simulink model "mpc_onlineHorizons"  (R2023a)
settings: Solver=ode23s  StartTime=0.0  StopTime=10  RelTol=1e-3
values from neighbouring files (symbols this model uses):
  r0 = -0.7    [RunTimeHorizonAdjustment1.m]
  x0 = [op_report.States(1).x;op_report.States(2).x]    [RunTimeHorizonAdjustment1.m]
  y0 = op_report.Outputs.y    [RunTimeHorizonAdjustment1.m]
libraries: mpclib x1
settings Model: ExtModeTrigMode=oneshot  Creator=The MathWorks, Inc.  LastModifiedBy=The MathWorks, Inc.
settings SolverCC: AlgebraicLoopSolver=TrustRegion
settings DataIOCC: SaveFormat=Array  ReturnWorkspaceOutputs=off  SignalLoggingName=sigsOut
settings OptimizationCC: BooleanDataType=off  ExpressionDepthLimit=2147483647  InitFltsAndDblsToZero=on  LifeSpan=inf
settings DebuggingCC: UnderspecifiedInitializationDetection=Classic  MergeDetectMultiDrivingBlocksExec=none  CheckExecutionContextPreStartOutputMsg=on  SignalResolutionControl=TryResolveAllWithWarning  MultiTaskDSMMsg=warning  MultiTaskCondExecSysMsg=none  IntegerOverflowMsg=none  FcnCallInpInsideContextMsg=warning  UnconnectedInputMsg=warning  UnconnectedOutputMsg=warning  UnconnectedLineMsg=warning  StateNameClashWarn=warning  SFUnexpectedBacktrackingDiag=warning  SFNoUnconditionalDefaultTransitionDiag=warning  SFExecutionAtInitializationDiag=none  IntegerSaturationMsg=none  ArithmeticOperatorsInVariantConditions=warning
settings HardwareCC: ProdBitPerPointer=32  ProdBitPerSizeT=32  ProdBitPerPtrDiffT=32  ProdLargestAtomicFloat=None  ProdIntDivRoundTo=Undefined  ProdEndianess=Unspecified  ProdWordSize=32  ProdHWDeviceType=32-bit Generic  TargetUnknown=on
settings ModelReferenceCC: EnableRefExpFcnMdlSchedulingChecks=on  PropagateSignalLabelsOutOfModel=off
settings SFSimCC: SimUseLocalCustomCode=off  CustomCodeUndefinedFunction=UseInterfaceOnly
settings RTWCC: RTWUseLocalCustomCode=off
settings CodeAppCC: StateflowObjectComments=on
settings GRTTargetCC: TargetLangStandard=C89/C90 (ANSI)  CombineOutputUpdateFcns=off  GRTInterface=on
settings ConfigComp: CovMetricSettings=dw  CovSaveCumulativeToWorkspaceVar=on  CovSaveSingleToWorkspaceVar=on  CovExternalEMLEnable=off  CovSFcnEnable=off

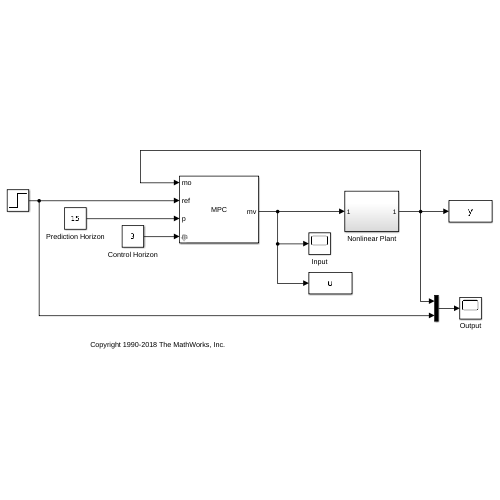
[thumbnail: Simulink's stored preview of the top-level diagram]
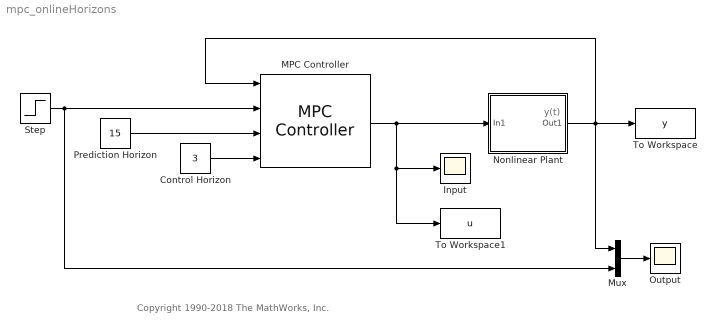
== system mpc_onlineHorizons ==
  note: y(t)
  note: Copyright 1990-2018 The MathWorks, Inc.
  Control Horizon : Constant  Value=3
  Input : Scope
  MPC Controller : mpclib/MPC Controller  mpcobj=mpcobj  x0=[]  is_multiple=0  enable_value=0  return_u0=off  updateMPCinCallerWorkspace=on  md_inport=off  mv_inport=off  uref_inport=off  return_cost=off  return_mvseq=off  return_qpstatus=off  return_xseq=off  return_state=off  return_ovseq=off  state_inport=off  umin_inport=off  umax_inport=off  ymin_inport=off  ymax_inport=off  cc_inport=off  ywt_inport=off  uwt_inport=off  duwt_inport=off  rhoeps_inport=off  pm_inport=on  MaximumP=50  HorizonChoice=VariableHorizon  n_ts=0.1  n_p=50  n_mv=1  n_md=0  n_ud=0  n_mo=1  n_uo=0  BlockDataType=double  SampleTimeInherited=off  switch_inport=off
  Mux : Mux  Inputs=2
  Nonlinear Plant : Subsystem
  Output : Scope
  Prediction Horizon : Constant  Value=15
  Step : Step  Before=y0  After=r0  SampleTime=0
  To Workspace : ToWorkspace  VariableName=y  SaveFormat=Structure With Time  SampleTime=-1
      settings: MaxDataPoints=Inf
  To Workspace1 : ToWorkspace  VariableName=u  SaveFormat=Structure With Time  SampleTime=-1
      settings: MaxDataPoints=Inf
  wires:
  MPC Controller/1 -> To Workspace1/1, Input/1, Nonlinear Plant/1(In1)
  Mux/1 -> Output/1
  Step/1 -> MPC Controller/2, Mux/2
  Nonlinear Plant/1(Out1) -> To Workspace/1, Mux/1, MPC Controller/1
  Prediction Horizon/1 -> MPC Controller/3
  Control Horizon/1 -> MPC Controller/4

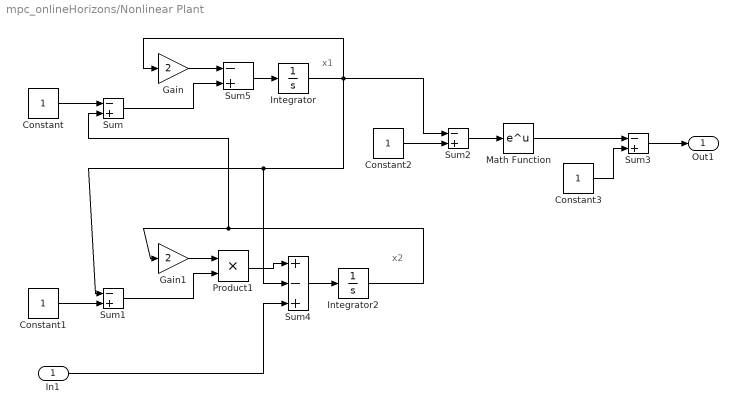
== system mpc_onlineHorizons/Nonlinear Plant ==
  note: x1
  note: x2
  In1 : Inport
  Constant{,1..3} (4 alike) : Constant
  Gain : Gain  Gain=2  SaturateOnIntegerOverflow=on  OutDataTypeStr=Inherit: Same as input  ParamDataTypeStr=Inherit: Same as input
  Gain1 : Gain  Gain=2  SaturateOnIntegerOverflow=on  OutDataTypeStr=Inherit: Same as input  ParamDataTypeStr=Inherit: Same as input
  Integrator : Integrator  InitialCondition=x0(1)  UpperSaturationLimit=Inf  LowerSaturationLimit=-Inf
  Integrator2 : Integrator  InitialCondition=x0(2)  UpperSaturationLimit=Inf  LowerSaturationLimit=-Inf
  Math Function : Math  SignedPower=on
  Product1 : Product  InputSameDT=on  SaturateOnIntegerOverflow=on  OutDataTypeStr=Inherit: Same as first input
  Sum{,1..3,5} (5 alike) : Sum  Inputs=-+  InputSameDT=on  SaturateOnIntegerOverflow=on  OutDataTypeStr=Inherit: Same as first input
  Sum4 : Sum  Inputs=+-+  InputSameDT=on  SaturateOnIntegerOverflow=on  OutDataTypeStr=Inherit: Same as first input
  Out1 : Outport  VectorParamsAs1DForOutWhenUnconnected=off
  wires:
  Sum5/1 -> Integrator/1
  Gain/1 -> Sum5/1
  Integrator/1 -> Gain/1, Sum2/1, Sum1/1, Sum4/2
  Constant/1 -> Sum/1
  Sum/1 -> Sum5/2
  Gain1/1 -> Product1/1
  Sum1/1 -> Product1/2
  Constant1/1 -> Sum1/2
  Constant2/1 -> Sum2/2
  Sum2/1 -> Math Function/1
  Constant3/1 -> Sum3/2
  Math Function/1 -> Sum3/1
  Sum3/1 -> Out1/1
  Integrator2/1 -> Gain1/1, Sum/2
  Sum4/1 -> Integrator2/1
  Product1/1 -> Sum4/1
  In1/1 -> Sum4/3
